simulink model "Transformer_model"  (R2016a)
settings: Solver=ode23tb  StartTime=0.0  StopTime=1  MaxStep=1e-4  RelTol=1e-3
undefined symbols (not defined in the file): D1, Delta
libraries: powerlib x21, powerlib_meascontrol x13
settings Model: Creator=AT Once  LastModifiedBy=AT Once

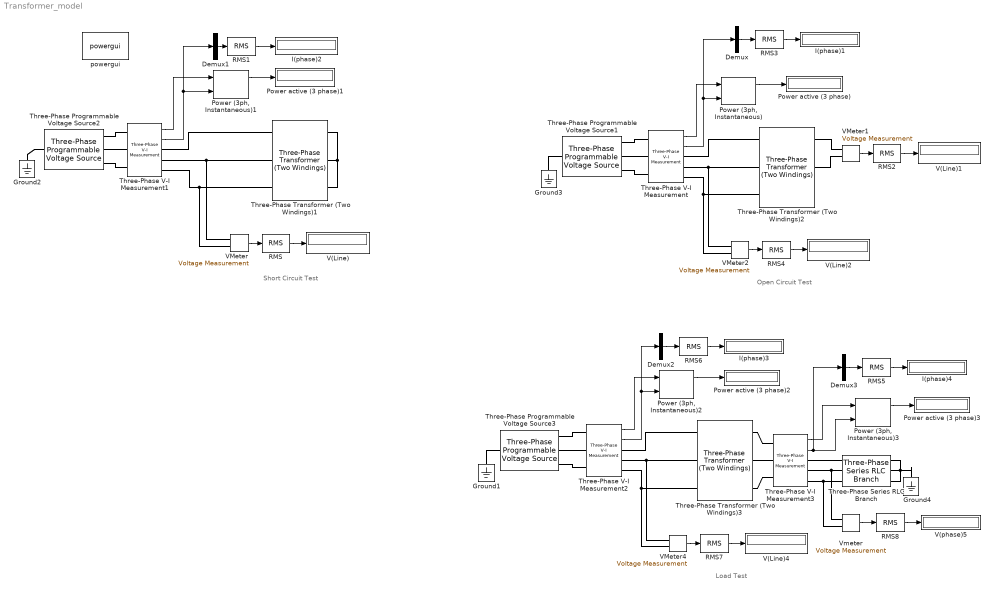
== system Transformer_model ==
  note: Short Circuit Test
  note: Open Circuit Test
  note: Load Test
  Demux{,1..3} (4 alike) : Demux  Outputs=1
  Ground{1..4} (4 alike) : powerlib/Elements/Ground  LConnTagsString=a
  I(phase){1..4} (4 alike) : Display
  Power (3ph, Instantaneous){,1..3} (4 alike) : powerlib_meascontrol/Measurements/Power (3ph, Instantaneous)
  Power active (3 phase){,1..3} (4 alike) : Display
  RMS{,1..8} (9 alike) : powerlib_meascontrol/Measurements/RMS  TrueRMS=on  Freq=50  RMSInit=0  Ts=0
  Three-Phase Programmable Voltage Source1 : powerlib/Electrical Sources/Three-Phase Programmable Voltage Source  PositiveSequence="[380  0 50]"  VariationEntity=None  VariationType=Table of time-amplitude pairs  VariationTypeAlt=Step  VariationStep=0.5  VariationRate=10  VariationMagnitude=0.3  VariationFrequency=2  VariationTiming=[1 2]  VariationPhaseA=off  Amplitudes=[1 0.8 1.2 1.0]  TimeValues=[0 0.1 0.15 0.2]  HarmonicGeneration=off  HarmonicA=[3 0.2 -25 0]  HarmonicB=[2 0.15 35 2]  Timing="[0.05  3]"  BusType=swing  Pref=0  Qref=0  Qmin=-inf  Qmax=inf
  Three-Phase Programmable Voltage Source2 : powerlib/Electrical Sources/Three-Phase Programmable Voltage Source  PositiveSequence="[10.4  0 50]"  VariationEntity=None  VariationType=Table of time-amplitude pairs  VariationTypeAlt=Step  VariationStep=0.5  VariationRate=10  VariationMagnitude=0.3  VariationFrequency=2  VariationTiming=[1 2]  VariationPhaseA=off  Amplitudes=[1 0.8 1.2 1.0]  TimeValues=[0 0.1 0.15 0.2]  HarmonicGeneration=off  HarmonicA=[3 0.2 -25 0]  HarmonicB=[2 0.15 35 2]  Timing="[0.05  3]"  BusType=swing  Pref=0  Qref=0  Qmin=-inf  Qmax=inf
  Three-Phase Programmable Voltage Source3 : powerlib/Electrical Sources/Three-Phase Programmable Voltage Source  PositiveSequence="[380  0 50]"  VariationEntity=None  VariationType=Table of time-amplitude pairs  VariationTypeAlt=Step  VariationStep=0.5  VariationRate=10  VariationMagnitude=0.3  VariationFrequency=2  VariationTiming=[1 2]  VariationPhaseA=off  Amplitudes=[1 0.8 1.2 1.0]  TimeValues=[0 0.1 0.15 0.2]  HarmonicGeneration=off  HarmonicA=[3 0.2 -25 0]  HarmonicB=[2 0.15 35 2]  Timing="[0.05  3]"  BusType=swing  Pref=0  Qref=0  Qmin=-inf  Qmax=inf
  Three-Phase Series RLC Branch : powerlib/Elements/Three-Phase Series RLC Branch  LConnTagsString=A|B|C  RConnTagsString=A|B|C  BranchType=R  Resistance=13  Inductance=1e-3  Capacitance=1e-6  Measurements=None
  Three-Phase Transformer (Two Windings)1 : powerlib/Elements/Three-Phase Transformer (Two Windings)  Winding1Connection=Y  Winding2Connection=Delta (D1)  CoreType=Three single-phase transformers  SetSaturation=off  Hysteresis=off  DataFile='hysteresis'  SetInitialFlux=off  Measurements=None  UNITS=SI  NominalPower=[ 250e6 , 50 ]  Winding1=[380 0 0]  Winding2=[220 0.5 1.1e-3]  Rm=3625  Lm=3.487  L0=0.5  Saturation=[0 0;0.66653 1910.3;277.72 2419.7]  InitialFluxes=[1273.5 -1273.5 1114.3]  MoreParameters=off  BreakLoop=off  DataType=on  TransfoNumber=1
  Three-Phase Transformer (Two Windings)2 : powerlib/Elements/Three-Phase Transformer (Two Windings)  Winding1Connection=Y  Winding2Connection=Delta (D1)  CoreType=Three single-phase transformers  SetSaturation=off  Hysteresis=off  DataFile='hysteresis'  SetInitialFlux=off  Measurements=None  UNITS=SI  NominalPower=[ 250e6 , 50 ]  Winding1=[380 0.0 0]  Winding2=[220 0.5 1.1e-3]  Rm=3625  Lm=3.487  L0=0.5  Saturation=[0 0;0.66653 1910.3;277.72 2419.7]  InitialFluxes=[1273.5 -1273.5 1114.3]  MoreParameters=off  BreakLoop=off  DataType=on  TransfoNumber=1
  Three-Phase Transformer (Two Windings)3 : powerlib/Elements/Three-Phase Transformer (Two Windings)  Winding1Connection=Y  Winding2Connection=Delta (D1)  CoreType=Three single-phase transformers  SetSaturation=off  Hysteresis=off  DataFile='hysteresis'  SetInitialFlux=off  Measurements=None  UNITS=SI  NominalPower=[ 250e6 , 50 ]  Winding1=[380 0.0 0]  Winding2=[230 0.5 1.1e-3]  Rm=3625  Lm=3.487  L0=0.5  Saturation=[0 0;0.66653 1910.3;277.72 2419.7]  InitialFluxes=[1273.5 -1273.5 1114.3]  MoreParameters=off  BreakLoop=off  DataType=on  TransfoNumber=1
  Three-Phase V-I Measurement{,1..3} (4 alike) : powerlib/Measurements/Three-Phase V-I Measurement  VoltageMeasurement=phase-to-ground  SetLabelV=off  LabelV=Vabc  Vpu=off  VpuLL=off  CurrentMeasurement=yes  SetLabelI=off  LabelI=Iabc  Ipu=off  Pbase=100e6  Vbase=500e3  OutputType=Complex  PhasorSimulation=off  PSBequivalent=0
  V(Line){,1..2,4} (4 alike) : Display
  V(phase)5 : Display
  VMeter{,1..2,4} (4 alike) : powerlib/Measurements/Voltage Measurement  PhasorSimulation=off  OutputType=Complex  PSBequivalent=0
  Vmeter : powerlib/Measurements/Voltage Measurement  PhasorSimulation=off  OutputType=Complex  PSBequivalent=0
  powergui : powerlib/powergui  Priority=1  SimulationMode=Continuous  SolverType=Tustin/Backward Euler (TBE)  SampleTime=50e-6  frequency=60  SPID=off  DisableSnubberDevices=off  DisableRonSwitches=off  DisableVfSwitches=off  SwTol=0  DisplayEquations=off  Interpol=off  ExternalGateDelay=off  methode=off  Ts=10  FunctionMessages=off  echomessages=off  HookPort=off  EnableUseOfTLC=off  x0status=blocks  frequencyindice=50  Pbase=100e6  ErrMax=1e-4  Iterations=50  UnitsV=kV  UnitsW=MW  buscounter=0  RestoreLinks=warning  ResistiveCurrentMeasurement=off  Frange=[0:2:500]  Ylog=off  Xlog=on  ShowGrid=off  save=off  variable=ZData  structure=0  ZoomFFT=off  StartTime=0.0  cycles=1  DisplayStyle=1  fundamental=60  FreqAxis=off  MaxFrequency=1000  frequencyindicesteady=1  RmsSteady=1  display=off
  wires:
  VMeter/1 -> RMS/1
  RMS/1 -> V(Line)/1
  VMeter1/1 -> RMS2/1
  RMS2/1 -> V(Line)1/1
  VMeter2/1 -> RMS4/1
  RMS4/1 -> V(Line)2/1
  Three-Phase V-I Measurement/2 -> Demux/1, "Power (3ph, Instantaneous)"/2
  Three-Phase V-I Measurement/1 -> "Power (3ph, Instantaneous)"/1
  "Power (3ph, Instantaneous)"/1 -> Power active (3 phase)/1
  RMS3/1 -> I(phase)1/1
  Demux/1 -> RMS3/1
  "Power (3ph, Instantaneous)1"/1 -> Power active (3 phase)1/1
  RMS1/1 -> I(phase)2/1
  Demux1/1 -> RMS1/1
  Three-Phase V-I Measurement1/1 -> "Power (3ph, Instantaneous)1"/1
  Three-Phase V-I Measurement1/2 -> Demux1/1, "Power (3ph, Instantaneous)1"/2
  VMeter4/1 -> RMS7/1
  RMS7/1 -> V(Line)4/1
  Three-Phase V-I Measurement2/2 -> "Power (3ph, Instantaneous)2"/2, Demux2/1
  Three-Phase V-I Measurement2/1 -> "Power (3ph, Instantaneous)2"/1
  "Power (3ph, Instantaneous)2"/1 -> Power active (3 phase)2/1
  RMS6/1 -> I(phase)3/1
  Demux2/1 -> RMS6/1
  "Power (3ph, Instantaneous)3"/1 -> Power active (3 phase)3/1
  RMS5/1 -> I(phase)4/1
  Demux3/1 -> RMS5/1
  Three-Phase V-I Measurement3/2 -> Demux3/1, "Power (3ph, Instantaneous)3"/2
  Three-Phase V-I Measurement3/1 -> "Power (3ph, Instantaneous)3"/1
  RMS8/1 -> V(phase)5/1
  Vmeter/1 -> RMS8/1
  connections:
  Three-Phase Transformer (Two Windings)1/RConn3 -- Three-Phase Transformer (Two Windings)1/RConn2 -- Three-Phase Transformer (Two Windings)1/RConn1
  VMeter2/LConn1 -- Three-Phase V-I Measurement/RConn2 -- Three-Phase Transformer (Two Windings)2/LConn2
  VMeter2/LConn2 -- Three-Phase V-I Measurement/RConn3 -- Three-Phase Transformer (Two Windings)2/LConn3
  VMeter1/LConn1 -- Three-Phase Transformer (Two Windings)2/RConn1
  VMeter1/LConn2 -- Three-Phase Transformer (Two Windings)2/RConn2
  Three-Phase V-I Measurement/RConn1 -- Three-Phase Transformer (Two Windings)2/LConn1
  Three-Phase Programmable Voltage Source2/RConn2 -- Three-Phase V-I Measurement1/LConn2
  Three-Phase Programmable Voltage Source2/RConn1 -- Three-Phase V-I Measurement1/LConn1
  Three-Phase Programmable Voltage Source2/RConn3 -- Three-Phase V-I Measurement1/LConn3
  Three-Phase V-I Measurement1/RConn3 -- VMeter/LConn2 -- Three-Phase Transformer (Two Windings)1/LConn3
  Three-Phase V-I Measurement1/RConn2 -- VMeter/LConn1 -- Three-Phase Transformer (Two Windings)1/LConn2
  Three-Phase V-I Measurement1/RConn1 -- Three-Phase Transformer (Two Windings)1/LConn1
  Three-Phase Programmable Voltage Source2/LConn1 -- Ground2/LConn1
  Three-Phase Programmable Voltage Source1/LConn1 -- Ground3/LConn1
  Three-Phase Programmable Voltage Source1/RConn1 -- Three-Phase V-I Measurement/LConn1
  Three-Phase Programmable Voltage Source1/RConn2 -- Three-Phase V-I Measurement/LConn2
  Three-Phase Programmable Voltage Source1/RConn3 -- Three-Phase V-I Measurement/LConn3
  VMeter4/LConn1 -- Three-Phase V-I Measurement2/RConn2 -- Three-Phase Transformer (Two Windings)3/LConn2
  VMeter4/LConn2 -- Three-Phase V-I Measurement2/RConn3 -- Three-Phase Transformer (Two Windings)3/LConn3
  Three-Phase Programmable Voltage Source3/RConn3 -- Three-Phase V-I Measurement2/LConn3
  Three-Phase Programmable Voltage Source3/RConn1 -- Three-Phase V-I Measurement2/LConn1
  Three-Phase Programmable Voltage Source3/RConn2 -- Three-Phase V-I Measurement2/LConn2
  Three-Phase Programmable Voltage Source3/LConn1 -- Ground1/LConn1
  Three-Phase V-I Measurement2/RConn1 -- Three-Phase Transformer (Two Windings)3/LConn1
  Three-Phase V-I Measurement3/LConn1 -- Three-Phase Transformer (Two Windings)3/RConn1
  Three-Phase V-I Measurement3/LConn2 -- Three-Phase Transformer (Two Windings)3/RConn2
  Three-Phase V-I Measurement3/LConn3 -- Three-Phase Transformer (Two Windings)3/RConn3
  Three-Phase Series RLC Branch/RConn1 -- Ground4/LConn1 -- Three-Phase Series RLC Branch/RConn3 -- Three-Phase Series RLC Branch/RConn2
  Three-Phase V-I Measurement3/RConn1 -- Three-Phase Series RLC Branch/LConn1
  Three-Phase V-I Measurement3/RConn2 -- Vmeter/LConn1 -- Three-Phase Series RLC Branch/LConn2
  Three-Phase V-I Measurement3/RConn3 -- Vmeter/LConn2 -- Three-Phase Series RLC Branch/LConn3
